simulink model "HW5_LQG"  (R2020a)
settings: Solver=ode1  StartTime=0.0  StopTime=inf  FixedStep=0.002  RelTol=1e-3  EnableMultiTasking=on
undefined symbols (not defined in the file): HIL, K, L, qc_get_step_size, sysd, T
libraries: quarc_library x3, simulink_extras x2, simulink x1
settings Model: ExtModeTrigDuration=5000  Creator=MLevis  LastModifiedBy=Jasper
settings DebuggingCC: UnderspecifiedInitializationDetection=Classic  MergeDetectMultiDrivingBlocksExec=none
settings ModelReferenceCC: PropagateSignalLabelsOutOfModel=off
settings SFSimCC: CustomCodeUndefinedFunction=UseInterfaceOnly

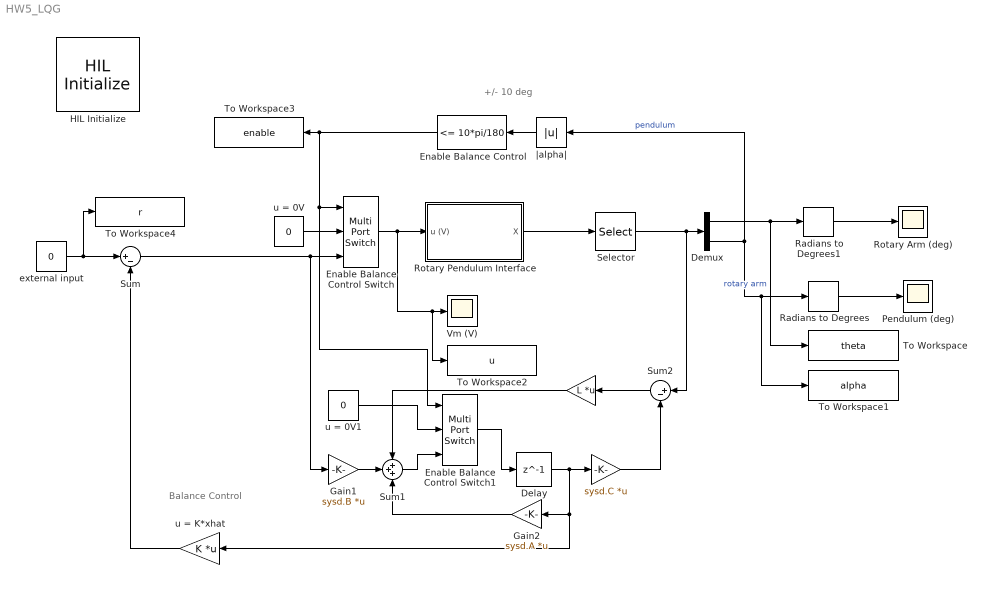
== system HW5_LQG ==
  note: +/- 10 deg
  note: Balance Control
  " " : Gain  Gain=sysd.C  Multiplication=Matrix(K*u)
  "  " : Gain  Gain=L  Multiplication=Matrix(K*u)
  Delay : Delay  DelayLength=1  SampleTime=T
  Demux : Demux  Outputs=2
  Enable Balance Control : simulink/Logic and Bit Operations/Compare To Constant  relop=<=  const=10*pi/180  OutDataTypeStr=uint8  ZeroCross=off
  Enable Balance Control Switch : MultiPortSwitch  DataPortOrder=Zero-based contiguous  Inputs=2  zeroidx=on
  Enable Balance Control Switch1 : MultiPortSwitch  DataPortOrder=Zero-based contiguous  Inputs=2  zeroidx=on
  Gain1 : Gain  Gain=sysd.B  Multiplication=Matrix(K*u)
  Gain2 : Gain  Gain=sysd.A  Multiplication=Matrix(K*u)
  HIL Initialize : quarc_library/Data Acquisition/Generic/Configuration/HIL Initialize  object_name=HIL-1  board_type=qube_servo2_usb  board_number=0@tcpip://localhost:18921  board_options=d0=digital;d1=digital;led=auto;update_rate=normal;decimation=1  exclusive=off  active=on  hardware_clocks=[0]  clock_modes=[]  initial_clock_frequencies=[]  set_clock_params_at_start=off  set_clock_params_at_switch_in=off  set_clock_frequencies_at_start=off  set_clock_frequencies_at_switch_in=off  analog_input_channels=[0]  analog_input_configurations=[]  analog_input_maximums=3  analog_input_minimums=-3  set_analog_input_params_at_start=off  set_analog_input_params_at_switch_in=off  analog_output_channels=[0]  analog_output_maximums=15  analog_output_minimums=-15  initial_analog_outputs=[0]  final_analog_outputs=[0]  watchdog_analog_outputs=0  set_analog_output_params_at_start=off  set_analog_output_params_at_switch_in=off  set_analog_outputs_at_start=on  set_analog_outputs_at_switch_in=off  set_analog_outputs_at_terminate=on  set_analog_outputs_at_switch_out=off  set_analog_outputs_on_watchdog=on  digital_input_channels=[]  digital_output_channels=[0]  digital_output_configuration=[]  initial_digital_outputs=[1]  final_digital_outputs=[0]  watchdog_digital_outputs=[0]  set_digital_output_params_at_start=off  set_digital_output_params_at_switch_in=off  set_digital_outputs_at_start=on  set_digital_outputs_at_switch_in=off  set_digital_outputs_at_terminate=on  set_digital_outputs_at_switch_out=off  set_digital_outputs_on_watchdog=on  encoder_channels=[0:1]  quadrature=[4]  encoder_filter_frequency=[]  initial_encoder_counts=[0]  set_encoder_params_at_start=off  set_encoder_params_at_switch_in=off  set_encoder_counts_at_start=on  set_encoder_counts_at_switch_in=off  pwm_channels=[]  pwm_modes=[]  pwm_frequency=[]  pwm_configuration=[]  pwm_alignment=[]  pwm_polarity=[]  pwm_leading_deadband=[]  pwm_trailing_deadband=[]  initial_pwm_outputs=[]  final_pwm_outputs=[]  watchdog_pwm_outputs=[]  set_pwm_params_at_start=off  set_pwm_params_at_switch_in=off  set_pwm_outputs_at_start=off  set_pwm_outputs_at_switch_in=off  set_pwm_outputs_at_terminate=off  set_pwm_outputs_at_switch_out=off  set_pwm_outputs_on_watchdog=off  other_output_channels=[11000:11002]  initial_other_outputs=[0 1 0]  final_other_outputs=[1 0 0]  watchdog_other_outputs=[0 0 1]  set_other_outputs_at_start=on  set_other_outputs_at_switch_in=off  set_other_outputs_at_terminate=on  set_other_outputs_at_switch_out=off  set_other_outputs_on_watchdog=on
  Pendulum (deg) : Scope
  Radians to Degrees : simulink_extras/Transformations/Radians to Degrees
  Radians to Degrees1 : simulink_extras/Transformations/Radians to Degrees
  Rotary Arm (deg) : Scope
  Rotary Pendulum Interface : Subsystem
  Selector : Selector  InputPortWidth=4  IndexOptions=Index vector (dialog)  Indices=[1 2]  OutputSizes=1
  Sum : Sum  Inputs=|+-
  Sum1 : Sum  Inputs=+++
  Sum2 : Sum  Inputs=|+-
  To Workspace : ToWorkspace  VariableName=theta  SaveFormat=Timeseries  SampleTime=-1
  To Workspace1 : ToWorkspace  VariableName=alpha  SaveFormat=Timeseries  SampleTime=-1
  To Workspace2 : ToWorkspace  VariableName=u  SaveFormat=Timeseries  SampleTime=-1
  To Workspace3 : ToWorkspace  VariableName=enable  SaveFormat=Timeseries  SampleTime=-1
  To Workspace4 : ToWorkspace  VariableName=r  SaveFormat=Timeseries  SampleTime=-1
  Vm (V) : Scope
  external input : Constant  Value=0
  u = 0V : Constant  Value=0
  u = 0V1 : Constant  Value=0
  u = K*xhat : Gain  Gain=K  Multiplication=Matrix(K*u)
  |alpha| : Abs
  wires:
  |alpha|/1 -> Enable Balance Control/1
  Enable Balance Control/1 -> To Workspace3/1, Enable Balance Control Switch1/1, Enable Balance Control Switch/1
  Radians to Degrees/1 -> Pendulum (deg)/1
  Radians to Degrees1/1 -> Rotary Arm (deg)/1
  Enable Balance Control Switch/1 -> To Workspace2/1, Vm (V)/1, Rotary Pendulum Interface/1(u (V))
  u = 0V/1 -> Enable Balance Control Switch/2
  Rotary Pendulum Interface/1(X) -> Selector/1
  Selector/1 -> Sum2/1, Demux/1
  Demux/1 -> To Workspace/1, Radians to Degrees1/1  "rotary arm"
  Demux/2 -> To Workspace1/1, Radians to Degrees/1, |alpha|/1  "pendulum"
  u = K*xhat/1 -> Sum/2
  external input/1 -> To Workspace4/1, Sum/1
  Gain2/1 -> Sum1/3
  Sum/1 -> Gain1/1, Enable Balance Control Switch/3
  Delay/1 -> u = K*xhat/1, Gain2/1, " "/1
  " "/1 -> Sum2/2
  Sum2/1 -> "  "/1
  Gain1/1 -> Sum1/2
  "  "/1 -> Sum1/1
  u = 0V1/1 -> Enable Balance Control Switch1/2
  Sum1/1 -> Enable Balance Control Switch1/3
  Enable Balance Control Switch1/1 -> Delay/1

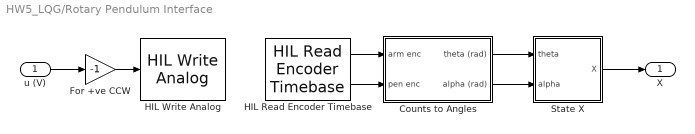
== system HW5_LQG/Rotary Pendulum Interface ==
  u (V) : Inport
  Counts to Angles : Subsystem
  For +ve CCW : Gain  Gain=-1
  HIL Read Encoder Timebase : quarc_library/Data Acquisition/Generic/Timebases/HIL Read Encoder Timebase  object_name=HIL-1  clock=0  channels=[0:1]  active=on  vector_output=off  data_type_mode=Inherit via back propagation  data_type=double  overflow_mode=Wait on overflow (for simulated cards only)  samples_in_buffer=1+0*max(ceil(1/qc_get_step_size), 1)
  HIL Write Analog : quarc_library/Data Acquisition/Generic/Immediate I//O/HIL Write Analog  object_name=HIL-1  channels=0  sample_time=-1  active=on  vector_input=off
  State X : Subsystem
  X : Outport  VectorParamsAs1DForOutWhenUnconnected=off
  wires:
  u (V)/1 -> For +ve CCW/1
  HIL Read Encoder Timebase/2 -> Counts to Angles/2(pen enc)
  For +ve CCW/1 -> HIL Write Analog/1
  HIL Read Encoder Timebase/1 -> Counts to Angles/1(arm enc)
  Counts to Angles/2(alpha (rad)) -> State X/2(alpha)
  Counts to Angles/1(theta (rad)) -> State X/1(theta)
  State X/1(X) -> X/1

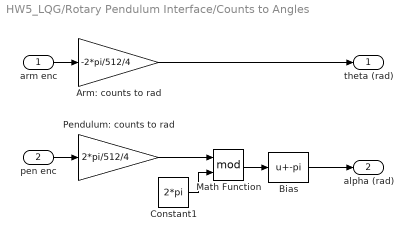
== system HW5_LQG/Rotary Pendulum Interface/Counts to Angles ==
  arm enc : Inport
  pen enc : Inport  Port=2
  Arm: counts to rad : Gain  Gain=-2*pi/512/4
  Bias : Bias  Bias=-pi
  Constant1 : Constant  Value=2*pi
  Math Function : Math  Operator=mod  SignedPower=on  SaturateOnIntegerOverflow=on
  Pendulum: counts to rad : Gain  Gain=2*pi/512/4
  theta (rad) : Outport  VectorParamsAs1DForOutWhenUnconnected=off
  alpha (rad) : Outport  Port=2  VectorParamsAs1DForOutWhenUnconnected=off
  wires:
  pen enc/1 -> Pendulum: counts to rad/1
  arm enc/1 -> Arm: counts to rad/1
  Math Function/1 -> Bias/1
  Constant1/1 -> Math Function/2
  Pendulum: counts to rad/1 -> Math Function/1
  Arm: counts to rad/1 -> theta (rad)/1
  Bias/1 -> alpha (rad)/1

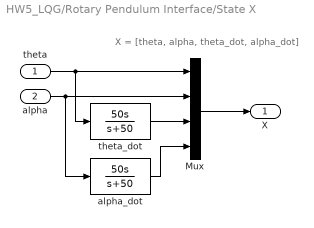
== system HW5_LQG/Rotary Pendulum Interface/State X ==
  note: X = [theta, alpha, theta_dot, alpha_dot]
  theta : Inport
  alpha : Inport  Port=2
  Mux : Mux
  alpha_dot : TransferFcn  Numerator=[50 0]  Denominator=[1 50]
  theta_dot : TransferFcn  Numerator=[50 0]  Denominator=[1 50]
  X : Outport  VectorParamsAs1DForOutWhenUnconnected=off
  wires:
  theta_dot/1 -> Mux/3
  alpha_dot/1 -> Mux/4
  alpha/1 -> Mux/2, alpha_dot/1
  Mux/1 -> X/1
  theta/1 -> Mux/1, theta_dot/1
